simulink model "VCMGCM1962020b_v2"  (R2020b)
settings: Solver=FixedStepDiscrete  StartTime=0.0  StopTime=10.0  FixedStep=0.005  RelTol=1e-3  EnableMultiTasking=on
PreLoadFcn:
  | try, model_open; catch, disp('Error occurred while executing model pre-load callback: model_open.m'); disp('Please assure that the MATLAB working directory is set to the model directory before opening.'); end
InitFcn:
  | try, model_open; catch, end
undefined symbols (not defined in the file): Bridge, GCM, H, raptor_get_param_eval, raptor_get_safe_string, raptor_xcp_function
libraries: Blocks_lib x1165, Raptor_lib x665, simulink x62, VCM_lib x5
(part 12 of 23)

== system VCMGCM1962020b_v2/Fgnd/Sensors/CAN/Battery/Status ==
  DiagEnbl : Inport
  Bus Creator : BusCreator  Inputs=11
  CANRxField1 : Blocks_lib/CANRxField  typ='double'  custom=off  custom_nam='---'  custom_units='---'
  CANRxField{3..10} (8 alike) : Blocks_lib/CANRxField  typ='boolean'  custom=off  custom_nam='---'  custom_units='---'
  CANRxField2 : Blocks_lib/CANRxField  typ='uint8'  custom=off  custom_nam='---'  custom_units='---'
  CANRxMsgStatus : Blocks_lib/CANRxMsgStatus  samptime=samptime  custom=off  custom_nam='---'  msgnam=Status
      link override CntrSat/Constant: OutDataTypeStr=uint32
      link override CntrSat/Constant1: OutDataTypeStr=uint32
      link override CntrSat/Relational Operator: Operator=>
      link override CntrSat/raptor_adjustment: dataType=uint32
  Header : Blocks_lib/Header  width=Landscape  addtext=''
  raptor_can_rxmsg : Raptor_lib/CAN/raptor_can_rxmsg  canDefinition=struct('dbcFile', 'eMatrix_Battery.dbc','message', 'Status','comment', '','signals', {{'ActivePacks','FaultID5','FaultID4','FaultID3','FaultID2','GFD','FaultID','PreContactor','PosContactor','NegContactor'}},'enabled', [ 1 1 1 1 1 1 1 1 1 1;],'scaled', [ 1 1 1 1 1 1 1 1 1 1;],'canBus', '''CAN1''','messageID', [ 277;],'idMask', [ 536870911;],'payloadMask', [],'payloadValue', [],'period', [ 0;],'mailbox', '''''','queueSize', [ 1;],'label', [ 0;],'ver', [ 2;],'showID', [ 0;],'showRaw', [ 0;],'fill', [ 0;],'editID', [ 0;],'signalOrder', [ 3;],'signalAscDes', [ 1;])  canBus='CAN1'  mailbox=''  payloadMask=[]  payloadValue=[]  idMask=hex2dec('1FFFFFFF')  queueSize=1  showID=0  label=0  fill=0  id=277  showRaw=0  showAge=1  signalOrder=3  signalInfo={{struct('Name', 'ActivePacks','Startbit', [ 0;],'SignalSize', [ 3;],'ByteOrder', 'LittleEndian','ValueType', 'UNSIGNED','Class', 'uint8','Signed', [ 0;],'Factor', [ 1;],'Offset', [ 0;],'Min', [ 0;],'Max', [ 0;],'Units', 'nmbr','Comment', 'Number of battery packs currently connected to the HV bus.','StartBit', [ 58;]),struct('Name', 'FaultID5','Startbit', [ 0;],'SignalSize', [ 8;],'ByteOrder', 'LittleEndian','ValueType', 'UNSIGNED','Class', 'uint8','Signed', [ 0;],'Factor', [ 1;],'Offset', [ 0;],'Min', [ 0;],'Max', [ 255;],'Units', 'Enum','Comment', '','StartBit', [ 48;]),struct('Name', 'FaultID4','Startbit', [ 0;],'SignalSize', [ 8;],'ByteOrder', 'LittleEndian','ValueType', 'UNSIGNED','Class', 'uint8','Signed', [ 0;],'Factor', [ 1;],'Offset', [ 0;],'Min', [ 0;],'Max', [ 255;],'Units', 'Enum','Comment', '','StartBit', [ 40;]),struct('Name', 'FaultID3','Startbit', [ 0;],'SignalSize', [ 8;],'ByteOrder', 'LittleEndian','ValueType', 'UNSIGNED','Class', 'uint8','Signed', [ 0;],'Factor', [ 1;],'Offset', [ 0;],'Min', [ 0;],'Max', [ 255;],'Units', 'Enum','Comment', '','StartBit', [ 32;]),struct('Name', 'FaultID2','Startbit', [ 0;],'SignalSize', [ 8;],'ByteOrder', 'LittleEndian','ValueType', 'UNSIGNED','Class', 'uint8','Signed', [ 0;],'Factor', [ 1;],'Offset', [ 0;],'Min', [ 0;],'Max', [ 255;],'Units', 'Enum','Comment', '','StartBit', [ 24;]),struct('Name', 'GFD','Startbit', [ 0;],'SignalSize', [ 16;],'ByteOrder', 'LittleEndian','ValueType', 'UNSIGNED','Class', 'uint16','Signed', [ 0;],'Factor', [ 1;],'Offset', [ 0;],'Min', [ 0;],'Max', [ 0;],'Units', 'Enum','Comment', '','StartBit', [ 0;]),struct('Name', 'FaultID','Startbit', [ 0;],'SignalSize', [ 8;],'ByteOrder', 'LittleEndian','ValueType', 'UNSIGNED','Class', 'uint8','Signed', [ 0;],'Factor', [ 1;],'Offset', [ 0;],'Min', [ 0;],'Max', [ 255;],'Units', 'Enum','Comment', '','StartBit', [ 16;]),struct('Name', 'PreContactor','Startbit', [ 0;],'SignalSize', [ 1;],'ByteOrder', 'LittleEndian','ValueType', 'UNSIGNED','Class', 'uint8','Signed', [ 0;],'Factor', [ 1;],'Offset', [ 0;],'Min', [ 0;],'Max', [ 0;],'Units', 'Bool','Comment', '0 = Open','StartBit', [ 63;]),struct('Name', 'PosContactor','Startbit', [ 0;],'SignalSize', [ 1;],'ByteOrder', 'LittleEndian','ValueType', 'UNSIGNED','Class', 'uint8','Signed', [ 0;],'Factor', [ 1;],'Offset', [ 0;],'Min', [ 0;],'Max', [ 0;],'Units', 'Bool','Comment', '0 = Open','StartBit', [ 62;]),struct('Name', 'NegContactor','Startbit', [ 0;],'SignalSize', [ 1;],'ByteOrder', 'LittleEndian','ValueType', 'UNSIGNED','Class', 'uint8','Signed', [ 0;],'Factor', [ 1;],'Offset', [ 0;],'Min', [ 0;],'Max', [ 0;],'Units', 'Bool','Comment', '0 = Open','StartBit', [ 61;])}}
      settings: SourceProductName=Raptor
  Data : Outport  VectorParamsAs1DForOutWhenUnconnected=off
  wires:
  CANRxField5/1 -> Bus Creator/6
  raptor_can_rxmsg/6 -> CANRxField5/1  "Batt_FltD2"
  Bus Creator/1 -> Data/1  "Status"
  CANRxField2/1 -> Bus Creator/3
  CANRxField3/1 -> Bus Creator/4
  CANRxField4/1 -> Bus Creator/5
  raptor_can_rxmsg/2 -> CANRxField1/1  "Batt_NmbrPcksActv"
  raptor_can_rxmsg/3 -> CANRxField2/1  "Batt_FltD5"
  raptor_can_rxmsg/4 -> CANRxField3/1  "Batt_FltD4"
  raptor_can_rxmsg/5 -> CANRxField4/1  "Batt_FltD3"
  CANRxField1/1 -> Bus Creator/2
  CANRxMsgStatus/1 -> Bus Creator/1
  DiagEnbl/1 -> CANRxMsgStatus/1
  raptor_can_rxmsg/1 -> CANRxMsgStatus/2  "Age"
  raptor_can_rxmsg/7 -> CANRxField6/1  "Batt_GFD"
  raptor_can_rxmsg/8 -> CANRxField7/1  "Batt_FltD"
  raptor_can_rxmsg/9 -> CANRxField8/1  "Batt_PreCntctr"
  raptor_can_rxmsg/10 -> CANRxField9/1  "Batt_PosCntctr"
  raptor_can_rxmsg/11 -> CANRxField10/1  "Batt_NegCntctr"
  CANRxField6/1 -> Bus Creator/7
  CANRxField7/1 -> Bus Creator/8
  CANRxField8/1 -> Bus Creator/9
  CANRxField9/1 -> Bus Creator/10
  CANRxField10/1 -> Bus Creator/11

== system VCMGCM1962020b_v2/Fgnd/Sensors/CAN/CCS Interface/CCSEVSE_ChargeParameters1 ==
  DiagEnbl : Inport
  Bus Creator : BusCreator  Inputs=5
  CANRxField{,1..3} (4 alike) : Blocks_lib/CANRxField  typ='double'  custom=on  custom_nam=[nam '---']  custom_units='---'
  CANRxMsgStatus : Blocks_lib/CANRxMsgStatus  samptime=samptime  custom=on  custom_nam=[nam '---']  msgnam=CCSEVSE_ChargeParameters1
  Header : Blocks_lib/Header  width=Landscape  addtext=''
  raptor_can_rxmsg : Raptor_lib/CAN/raptor_can_rxmsg  canDefinition=struct('dbcFile', 'm2iev-api.dbc','message', 'EVSE_ChargeParameters1','comment', 'EVSE_ChargeParameters1','signals', {{'EVSEMaximumCurrentLimit','EVSEMaximumVoltageLimit','EVSEMaximumPowerLimit','EVSEEnergyToBeDelivered'}},'enabled', [ 1 1 1 1;],'canBus', 'bus','messageID', [ 514;],'idMask', [ 2047;],'payloadMask', [],'payloadValue', [],'period', [ 0;],'mailbox', '''''','queueSize', [ 1;],'label', [ 1;],'ver', [ 2;],'showID', [ 0;],'showRaw', [ 0;],'fill', [ 0;],'editID', [ 0;],'signalOrder', [ 3;])  canBus=bus  mailbox=''  payloadMask=[]  payloadValue=[]  idMask=hex2dec('7FF')  queueSize=1  showID=0  label=1  fill=0  id=514  showRaw=0  showAge=1  signalOrder=3  signalInfo={{struct('Name', 'EVSEMaximumCurrentLimit','Startbit', [ 0;],'SignalSize', [ 16;],'ByteOrder', 'LittleEndian','ValueType', 'SIGNED','Class', 'int16','Signed', [ 1;],'Factor', [ 0.05;],'Offset', [ 0;],'Min', [ -1638.4;],'Max', [ 1638.35;],'Units', 'A','Comment', 'Maximim current EVSE is able to supply','StartBit', [ 0;]),struct('Name', 'EVSEMaximumVoltageLimit','Startbit', [ 0;],'SignalSize', [ 16;],'ByteOrder', 'LittleEndian','ValueType', 'UNSIGNED','Class', 'uint16','Signed', [ 0;],'Factor', [ 0.05;],'Offset', [ 0;],'Min', [ 0;],'Max', [ 3276.75;],'Units', 'V','Comment', 'Maximim voltage EVSE is able to supply','StartBit', [ 16;]),struct('Name', 'EVSEMaximumPowerLimit','Startbit', [ 0;],'SignalSize', [ 16;],'ByteOrder', 'LittleEndian','ValueType', 'UNSIGNED','Class', 'uint16','Signed', [ 0;],'Factor', [ 0.05;],'Offset', [ 0;],'Min', [ 0;],'Max', [ 3276.75;],'Units', 'kW','Comment', 'Maximum power EVSE is able to supply','StartBit', [ 32;]),struct('Name', 'EVSEEnergyToBeDelivered','Startbit', [ 0;],'SignalSize', [ 16;],'ByteOrder', 'LittleEndian','ValueType', 'UNSIGNED','Class', 'uint16','Signed', [ 0;],'Factor', [ 0.05;],'Offset', [ 0;],'Min', [ 0;],'Max', [ 3276.75;],'Units', 'kWh','Comment', 'Approximation of energy to be delivered','StartBit', [ 48;])}}
      settings: SourceProductName=Raptor
  Data : Outport  VectorParamsAs1DForOutWhenUnconnected=off
  wires:
  Bus Creator/1 -> Data/1  "MsgName"
  raptor_can_rxmsg/2 -> CANRxField/1  "EVSEMaximumCurrentLimit"
  raptor_can_rxmsg/3 -> CANRxField1/1  "EVSEMaximumVoltageLimit"
  raptor_can_rxmsg/4 -> CANRxField2/1  "EVSEMaximumPowerLimit"
  raptor_can_rxmsg/5 -> CANRxField3/1  "EVSEEnergyToBeDelivered"
  CANRxField3/1 -> Bus Creator/5
  CANRxField2/1 -> Bus Creator/4
  CANRxField1/1 -> Bus Creator/3
  CANRxField/1 -> Bus Creator/2
  CANRxMsgStatus/1 -> Bus Creator/1
  DiagEnbl/1 -> CANRxMsgStatus/1
  raptor_can_rxmsg/1 -> CANRxMsgStatus/2  "Age"

== system VCMGCM1962020b_v2/Fgnd/Sensors/CAN/CCS Interface/CCSEVSE_ChargeParameters2 ==
  DiagEnbl : Inport
  Bus Creator : BusCreator  Inputs=5
  CANRxField{,1..3} (4 alike) : Blocks_lib/CANRxField  typ='double'  custom=on  custom_nam=[nam '---']  custom_units='---'
  CANRxMsgStatus : Blocks_lib/CANRxMsgStatus  samptime=samptime  custom=on  custom_nam=[nam '---']  msgnam=CCSEVSE_ChargeParameters2
  Header : Blocks_lib/Header  width=Landscape  addtext=''
  raptor_can_rxmsg : Raptor_lib/CAN/raptor_can_rxmsg  canDefinition=struct('dbcFile', 'm2iev-api.dbc','message', 'EVSE_ChargeParameters2','comment', 'EVSE_ChargeParameters2','signals', {{'EVSEMinimumCurrentLimit','EVSEMinimumVoltageLimit','EVSECurrentRegulationTolerance','EVSEPeakCurrentRipple'}},'enabled', [ 1 1 1 1;],'canBus', 'bus','messageID', [ 515;],'idMask', [ 2047;],'payloadMask', [],'payloadValue', [],'period', [ 0;],'mailbox', '''''','queueSize', [ 1;],'label', [ 1;],'ver', [ 2;],'showID', [ 0;],'showRaw', [ 0;],'fill', [ 0;],'editID', [ 0;],'signalOrder', [ 3;])  canBus=bus  mailbox=''  payloadMask=[]  payloadValue=[]  idMask=hex2dec('7FF')  queueSize=1  showID=0  label=1  fill=0  id=515  showRaw=0  showAge=1  signalOrder=3  signalInfo={{struct('Name', 'EVSEMinimumCurrentLimit','Startbit', [ 0;],'SignalSize', [ 16;],'ByteOrder', 'LittleEndian','ValueType', 'SIGNED','Class', 'int16','Signed', [ 1;],'Factor', [ 0.05;],'Offset', [ 0;],'Min', [ -1638.4;],'Max', [ 1638.35;],'Units', 'A','Comment', 'Minimum current EVSE is able to supply','StartBit', [ 0;]),struct('Name', 'EVSEMinimumVoltageLimit','Startbit', [ 0;],'SignalSize', [ 16;],'ByteOrder', 'LittleEndian','ValueType', 'UNSIGNED','Class', 'uint16','Signed', [ 0;],'Factor', [ 0.05;],'Offset', [ 0;],'Min', [ 0;],'Max', [ 3276.75;],'Units', 'V','Comment', 'Minimum voltage EVSE is able to supply','StartBit', [ 16;]),struct('Name', 'EVSECurrentRegulationTolerance','Startbit', [ 0;],'SignalSize', [ 8;],'ByteOrder', 'LittleEndian','ValueType', 'UNSIGNED','Class', 'uint8','Signed', [ 0;],'Factor', [ 0.5;],'Offset', [ 0;],'Min', [ 0;],'Max', [ 127.5;],'Units', 'A','Comment', 'Tolerance of the current regulation','StartBit', [ 32;]),struct('Name', 'EVSEPeakCurrentRipple','Startbit', [ 0;],'SignalSize', [ 8;],'ByteOrder', 'LittleEndian','ValueType', 'UNSIGNED','Class', 'uint8','Signed', [ 0;],'Factor', [ 0.5;],'Offset', [ 0;],'Min', [ 0;],'Max', [ 127.5;],'Units', 'A','Comment', 'Peak current ripple that may occur on EVSE output','StartBit', [ 40;])}}
      settings: SourceProductName=Raptor
  Data : Outport  VectorParamsAs1DForOutWhenUnconnected=off
  wires:
  raptor_can_rxmsg/5 -> CANRxField3/1  "EVSEPeakCurrentRipple"
  raptor_can_rxmsg/4 -> CANRxField2/1  "EVSECurrentRegulationTolerance"
  raptor_can_rxmsg/3 -> CANRxField1/1  "EVSEMinimumVoltageLimit"
  raptor_can_rxmsg/2 -> CANRxField/1  "EVSEMinimumCurrentLimit"
  Bus Creator/1 -> Data/1  "MsgName"
  CANRxField3/1 -> Bus Creator/5
  CANRxField2/1 -> Bus Creator/4
  CANRxField1/1 -> Bus Creator/3
  CANRxField/1 -> Bus Creator/2
  CANRxMsgStatus/1 -> Bus Creator/1
  DiagEnbl/1 -> CANRxMsgStatus/1
  raptor_can_rxmsg/1 -> CANRxMsgStatus/2  "Age"

== system VCMGCM1962020b_v2/Fgnd/Sensors/CAN/CCS Interface/CCSEVSE_DC_ChargeInfo1 ==
  DiagEnbl : Inport
  Bus Creator : BusCreator  Inputs=9
  CANRxField : Blocks_lib/CANRxField  typ='uint8'  custom=on  custom_nam=[nam '---']  custom_units='---'
  CANRxField1 : Blocks_lib/CANRxField  typ='boolean'  custom=on  custom_nam=[nam '---']  custom_units='---'
  CANRxField2 : Blocks_lib/CANRxField  typ='boolean'  custom=on  custom_nam=[nam '---']  custom_units='---'
  CANRxField3 : Blocks_lib/CANRxField  typ='boolean'  custom=on  custom_nam=[nam '---']  custom_units='---'
  CANRxField4 : Blocks_lib/CANRxField  typ='uint8'  custom=on  custom_nam=[nam '---']  custom_units='---'
  CANRxField5 : Blocks_lib/CANRxField  typ='uint8'  custom=on  custom_nam=[nam '---']  custom_units='---'
  CANRxField6 : Blocks_lib/CANRxField  typ='double'  custom=on  custom_nam=[nam '---']  custom_units='---'
  CANRxField7 : Blocks_lib/CANRxField  typ='double'  custom=on  custom_nam=[nam '---']  custom_units='---'
  CANRxMsgStatus : Blocks_lib/CANRxMsgStatus  samptime=samptime  custom=on  custom_nam=[nam '---']  msgnam=CCSEVSE_DC_ChargeInfo1
  Header : Blocks_lib/Header  width=Landscape  addtext=''
  raptor_can_rxmsg : Raptor_lib/CAN/raptor_can_rxmsg  canDefinition=struct('dbcFile', 'm2iev-api.dbc','message', 'EVSE_DC_ChargeInfo1','comment', 'EVSE_DC_ChargeInfo1','signals', {{'ResponseCode','EVSECurrentLimitAchieved','EVSEVoltageLimitAchieved','EVSEPowerLimitAchieved','EVSEStatusCode','EVSEIsolationStatus','EVSEPresentVoltage','EVSEPresentCurrent'}},'enabled', [ 1 1 1 1 1 1 1 1;],'canBus', 'bus','messageID', [ 257;],'idMask', [ 2047;],'payloadMask', [],'payloadValue', [],'period', [ 0;],'mailbox', '''''','queueSize', [ 1;],'label', [ 1;],'ver', [ 2;],'showID', [ 0;],'showRaw', [ 0;],'fill', [ 0;],'editID', [ 0;],'signalOrder', [ 3;])  canBus=bus  mailbox=''  payloadMask=[]  payloadValue=[]  idMask=hex2dec('7FF')  queueSize=1  showID=0  label=1  fill=0  id=257  showRaw=0  showAge=1  signalOrder=3  signalInfo={{struct('Name', 'ResponseCode','Startbit', [ 0;],'SignalSize', [ 5;],'ByteOrder', 'LittleEndian','ValueType', 'UNSIGNED','Class', 'uint8','Signed', [ 0;],'Factor', [ 1;],'Offset', [ 0;],'Min', [ 0;],'Max', [ 26;],'Units', 'Enum','Comment', 'Response code from EVSE','StartBit', [ 0;]),struct('Name', 'EVSECurrentLimitAchieved','Startbit', [ 0;],'SignalSize', [ 1;],'ByteOrder', 'LittleEndian','ValueType', 'UNSIGNED','Class', 'uint8','Signed', [ 0;],'Factor', [ 1;],'Offset', [ 0;],'Min', [ 0;],'Max', [ 1;],'Units', 'Boolean','Comment', 'Indicator that EVSE is in current limiting mode','StartBit', [ 5;]),struct('Name', 'EVSEVoltageLimitAchieved','Startbit', [ 0;],'SignalSize', [ 1;],'ByteOrder', 'LittleEndian','ValueType', 'UNSIGNED','Class', 'uint8','Signed', [ 0;],'Factor', [ 1;],'Offset', [ 0;],'Min', [ 0;],'Max', [ 1;],'Units', 'Boolean','Comment', 'Indicator that EVSE is in voltage limiting mode','StartBit', [ 6;]),struct('Name', 'EVSEPowerLimitAchieved','Startbit', [ 0;],'SignalSize', [ 1;],'ByteOrder', 'LittleEndian','ValueType', 'UNSIGNED','Class', 'uint8','Signed', [ 0;],'Factor', [ 1;],'Offset', [ 0;],'Min', [ 0;],'Max', [ 1;],'Units', 'Boolean','Comment', 'Indicator that EVSE is in power limiting mode','StartBit', [ 7;]),struct('Name', 'EVSEStatusCode','Startbit', [ 0;],'SignalSize', [ 4;],'ByteOrder', 'LittleEndian','ValueType', 'UNSIGNED','Class', 'uint8','Signed', [ 0;],'Factor', [ 1;],'Offset', [ 0;],'Min', [ 0;],'Max', [ 11;],'Units', 'Enum','Comment', 'Status code reported by EVSE','StartBit', [ 8;]),struct('Name', 'EVSEIsolationStatus','Startbit', [ 0;],'SignalSize', [ 2;],'ByteOrder', 'LittleEndian','ValueType', 'UNSIGNED','Class', 'uint8','Signed', [ 0;],'Factor', [ 1;],'Offset', [ 0;],'Min', [ 0;],'Max', [ 3;],'Units', 'Enum','Comment', 'Isolation status detected by EVSE','StartBit', [ 12;]),struct('Name', 'EVSEPresentVoltage','Startbit', [ 0;],'SignalSize', [ 16;],'ByteOrder', 'LittleEndian','ValueType', 'UNSIGNED','Class', 'uint16','Signed', [ 0;],'Factor', [ 0.05;],'Offset', [ 0;],'Min', [ 0;],'Max', [ 3276.75;],'Units', 'V','Comment', 'Voltage supplied by EVSE (read on EVSE side)','StartBit', [ 16;]),struct('Name', 'EVSEPresentCurrent','Startbit', [ 0;],'SignalSize', [ 16;],'ByteOrder', 'LittleEndian','ValueType', 'SIGNED','Class', 'int16','Signed', [ 1;],'Factor', [ 0.05;],'Offset', [ 0;],'Min', [ -1638.4;],'Max', [ 1638.35;],'Units', 'A','Comment', 'Current supplied by EVSE (read on EVSE side)','StartBit', [ 32;])}}
      settings: SourceProductName=Raptor
  Data : Outport  VectorParamsAs1DForOutWhenUnconnected=off
  wires:
  raptor_can_rxmsg/6 -> CANRxField4/1  "EVSEStatusCode"
  raptor_can_rxmsg/5 -> CANRxField3/1  "EVSEPowerLimitAchieved"
  raptor_can_rxmsg/4 -> CANRxField2/1  "EVSEVoltageLimitAchieved"
  raptor_can_rxmsg/3 -> CANRxField1/1  "EVSECurrentLimitAchieved"
  raptor_can_rxmsg/2 -> CANRxField/1  "ResponseCode"
  Bus Creator/1 -> Data/1  "MsgName"
  raptor_can_rxmsg/7 -> CANRxField5/1  "EVSEIsolationStatus"
  raptor_can_rxmsg/8 -> CANRxField6/1  "EVSEPresentVoltage"
  raptor_can_rxmsg/9 -> CANRxField7/1  "EVSEPresentCurrent"
  CANRxField7/1 -> Bus Creator/9
  CANRxField6/1 -> Bus Creator/8
  CANRxField5/1 -> Bus Creator/7
  CANRxField4/1 -> Bus Creator/6
  CANRxField3/1 -> Bus Creator/5
  CANRxField2/1 -> Bus Creator/4
  CANRxField1/1 -> Bus Creator/3
  CANRxField/1 -> Bus Creator/2
  CANRxMsgStatus/1 -> Bus Creator/1
  DiagEnbl/1 -> CANRxMsgStatus/1
  raptor_can_rxmsg/1 -> CANRxMsgStatus/2  "Age"

== system VCMGCM1962020b_v2/Fgnd/Sensors/CAN/CCS Interface/CCSM2IEV_Alerts ==
  DiagEnbl : Inport
  Bus Creator : BusCreator  Inputs=16
  CANRxField{,1..14} (15 alike) : Blocks_lib/CANRxField  typ='boolean'  custom=on  custom_nam=[nam '---']  custom_units='---'
  CANRxMsgStatus : Blocks_lib/CANRxMsgStatus  samptime=samptime  custom=on  custom_nam=[nam '---']  msgnam=CCSM2IEV_Alerts
  Header : Blocks_lib/Header  width=Landscape  addtext=''
  raptor_can_rxmsg : Raptor_lib/CAN/raptor_can_rxmsg  canDefinition=struct('dbcFile', 'm2iev-api.dbc','message', 'M2IEV_Alerts','comment', 'M2IEV_Alerts','signals', {{'TemperatureDC1HighAlarm','TemperatureDC1HighFault','TemperatureDC1LowAlarm','TemperatureDC1LowFault','TemperatureDC2HighAlarm','TemperatureDC2HighFault','TemperatureDC2LowAlarm','TemperatureDC2LowFault','TemperatureACFault','EmergencyStopFault','PilotFault','ProximityFault','CanRxFault','SocketLatchSensorFault','EvccError'}},'enabled', [ 1 1 1 1 1 1 1 1 1 1 1 1 1 1 1;],'canBus', 'bus','messageID', [ 260;],'idMask', [ 2047;],'payloadMask', [],'payloadValue', [],'period', [ 0;],'mailbox', '''''','queueSize', [ 1;],'label', [ 1;],'ver', [ 2;],'showID', [ 0;],'showRaw', [ 0;],'fill', [ 0;],'editID', [ 0;],'signalOrder', [ 3;],'signalAscDes', [ 1;])  canBus=bus  mailbox=''  payloadMask=[]  payloadValue=[]  idMask=hex2dec('7FF')  queueSize=1  showID=0  label=1  fill=0  id=260  showRaw=0  showAge=1  signalOrder=3  signalInfo={{struct('Name', 'TemperatureDC1HighAlarm','Startbit', [ 0;],'SignalSize', [ 1;],'ByteOrder', 'LittleEndian','ValueType', 'UNSIGNED','Class', 'uint8','Signed', [ 0;],'Factor', [ 1;],'Offset', [ 0;],'Min', [ 0;],'Max', [ 1;],'Units', 'Boolean','Comment', 'Temperature on DC+ terminal >=80 degC','StartBit', [ 0;]),struct('Name', 'TemperatureDC1HighFault','Startbit', [ 0;],'SignalSize', [ 1;],'ByteOrder', 'LittleEndian','ValueType', 'UNSIGNED','Class', 'uint8','Signed', [ 0;],'Factor', [ 1;],'Offset', [ 0;],'Min', [ 0;],'Max', [ 1;],'Units', 'Boolean','Comment', 'Temperature on DC+ terminal >=90 degC','StartBit', [ 1;]),struct('Name', 'TemperatureDC1LowAlarm','Startbit', [ 0;],'SignalSize', [ 1;],'ByteOrder', 'LittleEndian','ValueType', 'UNSIGNED','Class', 'uint8','Signed', [ 0;],'Factor', [ 1;],'Offset', [ 0;],'Min', [ 0;],'Max', [ 1;],'Units', 'Boolean','Comment', 'Temperature on DC+ terminal <=-20 degC','StartBit', [ 2;]),struct('Name', 'TemperatureDC1LowFault','Startbit', [ 0;],'SignalSize', [ 1;],'ByteOrder', 'LittleEndian','ValueType', 'UNSIGNED','Class', 'uint8','Signed', [ 0;],'Factor', [ 1;],'Offset', [ 0;],'Min', [ 0;],'Max', [ 1;],'Units', 'Boolean','Comment', 'Temperature on DC+ terminal <=-30 degC','StartBit', [ 3;]),struct('Name', 'TemperatureDC2HighAlarm','Startbit', [ 0;],'SignalSize', [ 1;],'ByteOrder', 'LittleEndian','ValueType', 'UNSIGNED','Class', 'uint8','Signed', [ 0;],'Factor', [ 1;],'Offset', [ 0;],'Min', [ 0;],'Max', [ 1;],'Units', 'Boolean','Comment', 'Temperature on DC- terminal >=80 degC','StartBit', [ 4;]),struct('Name', 'TemperatureDC2HighFault','Startbit', [ 0;],'SignalSize', [ 1;],'ByteOrder', 'LittleEndian','ValueType', 'UNSIGNED','Class', 'uint8','Signed', [ 0;],'Factor', [ 1;],'Offset', [ 0;],'Min', [ 0;],'Max', [ 1;],'Units', 'Boolean','Comment', 'Temperature on DC- terminal >=90 degC','StartBit', [ 5;]),struct('Name', 'TemperatureDC2LowAlarm','Startbit', [ 0;],'SignalSize', [ 1;],'ByteOrder', 'LittleEndian','ValueType', 'UNSIGNED','Class', 'uint8','Signed', [ 0;],'Factor', [ 1;],'Offset', [ 0;],'Min', [ 0;],'Max', [ 1;],'Units', 'Boolean','Comment', 'Temperature on DC- terminal <=-20 degC','StartBit', [ 6;]),struct('Name', 'TemperatureDC2LowFault','Startbit', [ 0;],'SignalSize', [ 1;],'ByteOrder', 'LittleEndian','ValueType', 'UNSIGNED','Class', 'uint8','Signed', [ 0;],'Factor', [ 1;],'Offset', [ 0;],'Min', [ 0;],'Max', [ 1;],'Units', 'Boolean','Comment', 'Temperature on DC- terminal <=-30 degC','StartBit', [ 7;]),struct('Name', 'TemperatureACFault','Startbit', [ 0;],'SignalSize', [ 1;],'ByteOrder', 'LittleEndian','ValueType', 'UNSIGNED','Class', 'uint8','Signed', [ 0;],'Factor', [ 1;],'Offset', [ 0;],'Min', [ 0;],'Max', [ 1;],'Units', 'Boolean','Comment', 'Temperature on AC terminals is too high','StartBit', [ 8;]),struct('Name', 'EmergencyStopFault','Startbit', [ 0;],'SignalSize', [ 1;],'ByteOrder', 'LittleEndian','ValueType', 'UNSIGNED','Class', 'uint8','Signed', [ 0;],'Factor', [ 1;],'Offset', [ 0;],'Min', [ 0;],'Max', [ 1;],'Units', 'Boolean','Comment', 'Emergency stop','StartBit', [ 9;]),struct('Name', 'PilotFault','Startbit', [ 0;],'SignalSize', [ 1;],'ByteOrder', 'LittleEndian','ValueType', 'UNSIGNED','Class', 'uint8','Signed', [ 0;],'Factor', [ 1;],'Offset', [ 0;],'Min', [ 0;],'Max', [ 1;],'Units', 'Boolean','Comment', 'Pilot fault','StartBit', [ 10;]),struct('Name', 'ProximityFault','Startbit', [ 0;],'SignalSize', [ 1;],'ByteOrder', 'LittleEndian','ValueType', 'UNSIGNED','Class', 'uint8','Signed', [ 0;],'Factor', [ 1;],'Offset', [ 0;],'Min', [ 0;],'Max', [ 1;],'Units', 'Boolean','Comment', 'Proximity fault','StartBit', [ 11;]),struct('Name', 'CanRxFault','Startbit', [ 0;],'SignalSize', [ 1;],'ByteOrder', 'LittleEndian','ValueType', 'UNSIGNED','Class', 'uint8','Signed', [ 0;],'Factor', [ 1;],'Offset', [ 0;],'Min', [ 0;],'Max', [ 1;],'Units', 'Boolean','Comment', 'Can Rx fault','StartBit', [ 12;]),struct('Name', 'SocketLatchSensorFault','Startbit', [ 0;],'SignalSize', [ 1;],'ByteOrder', 'LittleEndian','ValueType', 'UNSIGNED','Class', 'uint8','Signed', [ 0;],'Factor', [ 1;],'Offset', [ 0;],'Min', [ 0;],'Max', [ 1;],'Units', 'Boolean','Comment', 'Socket latch sensor fault','StartBit', [ 13;]),struct('Name', 'EvccError','Startbit', [ 0;],'SignalSize', [ 1;],'ByteOrder', 'LittleEndian','ValueType', 'UNSIGNED','Class', 'uint8','Signed', [ 0;],'Factor', [ 1;],'Offset', [ 0;],'Min', [ 0;],'Max', [ 1;],'Units', 'Boolean','Comment', 'Received EVCC error','StartBit', [ 14;])}}
      settings: SourceProductName=Raptor
  Data : Outport  VectorParamsAs1DForOutWhenUnconnected=off
  wires:
  raptor_can_rxmsg/10 -> CANRxField8/1  "TemperatureACFault"
  raptor_can_rxmsg/11 -> CANRxField9/1  "EmergencyStopFault"
  raptor_can_rxmsg/13 -> CANRxField11/1  "ProximityFault"
  raptor_can_rxmsg/12 -> CANRxField10/1  "PilotFault"
  raptor_can_rxmsg/16 -> CANRxField14/1  "EvccError"
  raptor_can_rxmsg/15 -> CANRxField13/1  "SocketLatchSensorFault"
  raptor_can_rxmsg/14 -> CANRxField12/1  "CanRxFault"
  raptor_can_rxmsg/6 -> CANRxField4/1  "TemperatureDC2HighAlarm"
  raptor_can_rxmsg/7 -> CANRxField5/1  "TemperatureDC2HighFault"
  raptor_can_rxmsg/9 -> CANRxField7/1  "TemperatureDC2LowFault"
  raptor_can_rxmsg/8 -> CANRxField6/1  "TemperatureDC2LowAlarm"
  raptor_can_rxmsg/4 -> CANRxField2/1  "TemperatureDC1LowAlarm"
  raptor_can_rxmsg/5 -> CANRxField3/1  "TemperatureDC1LowFault"
  raptor_can_rxmsg/3 -> CANRxField1/1  "TemperatureDC1HighFault"
  raptor_can_rxmsg/2 -> CANRxField/1  "TemperatureDC1HighAlarm"
  Bus Creator/1 -> Data/1  "MsgName"
  CANRxField11/1 -> Bus Creator/13
  CANRxField10/1 -> Bus Creator/12
  CANRxField12/1 -> Bus Creator/14
  CANRxField9/1 -> Bus Creator/11
  CANRxField13/1 -> Bus Creator/15
  CANRxField8/1 -> Bus Creator/10
  CANRxField14/1 -> Bus Creator/16
  CANRxField7/1 -> Bus Creator/9
  CANRxField6/1 -> Bus Creator/8
  CANRxField5/1 -> Bus Creator/7
  CANRxField4/1 -> Bus Creator/6
  CANRxField3/1 -> Bus Creator/5
  CANRxField2/1 -> Bus Creator/4
  CANRxField1/1 -> Bus Creator/3
  CANRxField/1 -> Bus Creator/2
  CANRxMsgStatus/1 -> Bus Creator/1
  DiagEnbl/1 -> CANRxMsgStatus/1
  raptor_can_rxmsg/1 -> CANRxMsgStatus/2  "Age"

== system VCMGCM1962020b_v2/Fgnd/Sensors/CAN/CCS Interface/CCSM2IEV_Command ==
  DiagEnbl : Inport
  Bus Creator : BusCreator  Inputs=8
  CANRxField{,1,5..6} (4 alike) : Blocks_lib/CANRxField  typ='uint8'  custom=on  custom_nam=[nam '---']  custom_units='---'
  CANRxField2 : Blocks_lib/CANRxField  typ='boolean'  custom=on  custom_nam=[nam '---']  custom_units='---'
  CANRxField3 : Blocks_lib/CANRxField  typ='boolean'  custom=on  custom_nam=[nam '---']  custom_units='---'
  CANRxField4 : Blocks_lib/CANRxField  typ='boolean'  custom=on  custom_nam=[nam '---']  custom_units='---'
  CANRxMsgStatus : Blocks_lib/CANRxMsgStatus  samptime=samptime  custom=on  custom_nam=[nam '---']  msgnam=CCSM2IEV_Command
  Header : Blocks_lib/Header  width=Landscape  addtext=''
  raptor_can_rxmsg : Raptor_lib/CAN/raptor_can_rxmsg  canDefinition=struct('dbcFile', 'm2iev-api.dbc','message', 'M2IEV_Command','comment', 'M2IEV_Command','signals', {{'CurrentState','ChargerType','AC_CloseContactorsRequest','DC_CloseContactorsRequest','PrechargeReady','SocketLockState','ErrorCode'}},'enabled', [ 1 1 1 1 1 1 1;],'canBus', 'bus','messageID', [ 129;],'idMask', [ 2047;],'payloadMask', [],'payloadValue', [],'period', [ 0;],'mailbox', '''''','queueSize', [ 1;],'label', [ 1;],'ver', [ 2;],'showID', [ 0;],'showRaw', [ 0;],'fill', [ 0;],'editID', [ 0;],'signalOrder', [ 3;])  canBus=bus  mailbox=''  payloadMask=[]  payloadValue=[]  idMask=hex2dec('7FF')  queueSize=1  showID=0  label=1  fill=0  id=129  showRaw=0  showAge=1  signalOrder=3  signalInfo={{struct('Name', 'CurrentState','Startbit', [ 0;],'SignalSize', [ 8;],'ByteOrder', 'LittleEndian','ValueType', 'UNSIGNED','Class', 'uint8','Signed', [ 0;],'Factor', [ 1;],'Offset', [ 0;],'Min', [ 0;],'Max', [ 255;],'Units', 'Enum','Comment', 'Current state of M2IEV module','StartBit', [ 0;]),struct('Name', 'ChargerType','Startbit', [ 0;],'SignalSize', [ 3;],'ByteOrder', 'LittleEndian','ValueType', 'UNSIGNED','Class', 'uint8','Signed', [ 0;],'Factor', [ 1;],'Offset', [ 0;],'Min', [ 0;],'Max', [ 3;],'Units', 'Enum','Comment', 'Type of the charger connected','StartBit', [ 8;]),struct('Name', 'AC_CloseContactorsRequest','Startbit', [ 0;],'SignalSize', [ 1;],'ByteOrder', 'LittleEndian','ValueType', 'UNSIGNED','Class', 'uint8','Signed', [ 0;],'Factor', [ 1;],'Offset', [ 0;],'Min', [ 0;],'Max', [ 1;],'Units', 'Boolean','Comment', 'Request to close AC contactors (i.e. request to start power transfer)','StartBit', [ 11;]),struct('Name', 'DC_CloseContactorsRequest','Startbit', [ 0;],'SignalSize', [ 1;],'ByteOrder', 'LittleEndian','ValueType', 'UNSIGNED','Class', 'uint8','Signed', [ 0;],'Factor', [ 1;],'Offset', [ 0;],'Min', [ 0;],'Max', [ 1;],'Units', 'Boolean','Comment', 'Request to close DC contactors (i.e. request to start power transfer)','StartBit', [ 12;]),struct('Name', 'PrechargeReady','Startbit', [ 0;],'SignalSize', [ 1;],'ByteOrder', 'LittleEndian','ValueType', 'UNSIGNED','Class', 'uint8','Signed', [ 0;],'Factor', [ 1;],'Offset', [ 0;],'Min', [ 0;],'Max', [ 1;],'Units', 'Boolean','Comment', 'Indicator that cable check has successfully passed and we are ready to start precharging (valid only in case of smart DC charging)','StartBit', [ 13;]),struct('Name', 'SocketLockState','Startbit', [ 0;],'SignalSize', [ 3;],'ByteOrder', 'LittleEndian','ValueType', 'UNSIGNED','Class', 'uint8','Signed', [ 0;],'Factor', [ 1;],'Offset', [ 0;],'Min', [ 0;],'Max', [ 5;],'Units', 'Enum','Comment', 'Current socket state','StartBit', [ 24;]),struct('Name', 'ErrorCode','Startbit', [ 0;],'SignalSize', [ 16;],'ByteOrder', 'LittleEndian','ValueType', 'UNSIGNED','Class', 'uint16','Signed', [ 0;],'Factor', [ 1;],'Offset', [ 0;],'Min', [ 0;],'Max', [ 65535;],'Units', 'Enum','Comment', 'Internal M2IEV or EVCC error code','StartBit', [ 32;])}}
      settings: SourceProductName=Raptor
  Data : Outport  VectorParamsAs1DForOutWhenUnconnected=off
  wires:
  raptor_can_rxmsg/6 -> CANRxField4/1  "PrechargeReady"
  raptor_can_rxmsg/5 -> CANRxField3/1  "DC_CloseContactorsRequest"
  raptor_can_rxmsg/4 -> CANRxField2/1  "AC_CloseContactorsRequest"
  raptor_can_rxmsg/3 -> CANRxField1/1  "ChargerType"
  raptor_can_rxmsg/2 -> CANRxField/1  "CurrentState"
  Bus Creator/1 -> Data/1  "MsgName"
  raptor_can_rxmsg/7 -> CANRxField5/1  "SocketLockState"
  raptor_can_rxmsg/8 -> CANRxField6/1  "ErrorCode"
  CANRxField6/1 -> Bus Creator/8
  CANRxField5/1 -> Bus Creator/7
  CANRxField4/1 -> Bus Creator/6
  CANRxField3/1 -> Bus Creator/5
  CANRxField2/1 -> Bus Creator/4
  CANRxField1/1 -> Bus Creator/3
  CANRxField/1 -> Bus Creator/2
  CANRxMsgStatus/1 -> Bus Creator/1
  DiagEnbl/1 -> CANRxMsgStatus/1
  raptor_can_rxmsg/1 -> CANRxMsgStatus/2  "Age"

== system VCMGCM1962020b_v2/Fgnd/Sensors/CAN/CCS Interface/CCSM2IEV_Info ==
  DiagEnbl : Inport
  Bus Creator : BusCreator  Inputs=5
  CANRxField : Blocks_lib/CANRxField  typ='uint8'  custom=on  custom_nam=[nam '---']  custom_units='---'
  CANRxField1 : Blocks_lib/CANRxField  typ='uint8'  custom=on  custom_nam=[nam '---']  custom_units='---'
  CANRxField2 : Blocks_lib/CANRxField  typ='double'  custom=on  custom_nam=[nam '---']  custom_units='---'
  CANRxField3 : Blocks_lib/CANRxField  typ='double'  custom=on  custom_nam=[nam '---']  custom_units='---'
  CANRxMsgStatus : Blocks_lib/CANRxMsgStatus  samptime=samptime  custom=on  custom_nam=[nam '---']  msgnam=CCSM2IEV_Info
  Header : Blocks_lib/Header  width=Landscape  addtext=''
  raptor_can_rxmsg : Raptor_lib/CAN/raptor_can_rxmsg  canDefinition=struct('dbcFile', 'm2iev-api.dbc','message', 'M2IEV_Info','comment', 'M2IEV_Info','signals', {{'PP_State','CP_State','CP_PWM','CP_Voltage'}},'enabled', [ 1 1 1 1;],'canBus', 'bus','messageID', [ 130;],'idMask', [ 2047;],'payloadMask', [],'payloadValue', [],'period', [ 0;],'mailbox', '''''','queueSize', [ 1;],'label', [ 1;],'ver', [ 2;],'showID', [ 0;],'showRaw', [ 0;],'fill', [ 0;],'editID', [ 0;],'signalOrder', [ 3;],'signalAscDes', [ 1;])  canBus=bus  mailbox=''  payloadMask=[]  payloadValue=[]  idMask=hex2dec('7FF')  queueSize=1  showID=0  label=1  fill=0  id=130  showRaw=0  showAge=1  signalOrder=3  signalInfo={{struct('Name', 'PP_State','Startbit', [ 0;],'SignalSize', [ 4;],'ByteOrder', 'LittleEndian','ValueType', 'UNSIGNED','Class', 'uint8','Signed', [ 0;],'Factor', [ 1;],'Offset', [ 0;],'Min', [ 0;],'Max', [ 7;],'Units', 'Enum','Comment', 'Current proximity state','StartBit', [ 0;]),struct('Name', 'CP_State','Startbit', [ 0;],'SignalSize', [ 4;],'ByteOrder', 'LittleEndian','ValueType', 'UNSIGNED','Class', 'uint8','Signed', [ 0;],'Factor', [ 1;],'Offset', [ 0;],'Min', [ 0;],'Max', [ 7;],'Units', 'Enum','Comment', 'Current control pilot state','StartBit', [ 4;]),struct('Name', 'CP_PWM','Startbit', [ 0;],'SignalSize', [ 8;],'ByteOrder', 'LittleEndian','ValueType', 'UNSIGNED','Class', 'uint8','Signed', [ 0;],'Factor', [ 1;],'Offset', [ 0;],'Min', [ 0;],'Max', [ 100;],'Units', '%','Comment', 'Current control pilot PWM duty ratio','StartBit', [ 8;]),struct('Name', 'CP_Voltage','Startbit', [ 0;],'SignalSize', [ 9;],'ByteOrder', 'LittleEndian','ValueType', 'SIGNED','Class', 'int16','Signed', [ 1;],'Factor', [ 0.1;],'Offset', [ 0;],'Min', [ -25.6;],'Max', [ 25.5;],'Units', 'V','Comment', 'Current voltage on control pilot line','StartBit', [ 16;])}}
      settings: SourceProductName=Raptor
  Data : Outport  VectorParamsAs1DForOutWhenUnconnected=off
  wires:
  raptor_can_rxmsg/5 -> CANRxField3/1  "CP_Voltage"
  raptor_can_rxmsg/4 -> CANRxField2/1  "CP_PWM"
  raptor_can_rxmsg/3 -> CANRxField1/1  "CP_State"
  raptor_can_rxmsg/2 -> CANRxField/1  "PP_State"
  Bus Creator/1 -> Data/1  "MsgName"
  CANRxField3/1 -> Bus Creator/5
  CANRxField2/1 -> Bus Creator/4
  CANRxField1/1 -> Bus Creator/3
  CANRxField/1 -> Bus Creator/2
  CANRxMsgStatus/1 -> Bus Creator/1
  DiagEnbl/1 -> CANRxMsgStatus/1
  raptor_can_rxmsg/1 -> CANRxMsgStatus/2  "Age"

== system VCMGCM1962020b_v2/Fgnd/Sensors/CAN/CCS Interface/CCSM2IEV_TemperatureInfo ==
  DiagEnbl : Inport
  Bus Creator : BusCreator  Inputs=4
  CANRxField : Blocks_lib/CANRxField  typ='double'  custom=on  custom_nam=[nam '---']  custom_units='---'
  CANRxField1 : Blocks_lib/CANRxField  typ='double'  custom=on  custom_nam=[nam '---']  custom_units='---'
  CANRxField2 : Blocks_lib/CANRxField  typ='double'  custom=on  custom_nam=[nam '---']  custom_units='---'
  CANRxMsgStatus : Blocks_lib/CANRxMsgStatus  samptime=samptime  custom=on  custom_nam=[nam '---']  msgnam=CCSM2IEV_TemperatureInfo
  Header : Blocks_lib/Header  width=Landscape  addtext=''
  raptor_can_rxmsg : Raptor_lib/CAN/raptor_can_rxmsg  canDefinition=struct('dbcFile', 'm2iev-api.dbc','message', 'M2IEV_TemperatureInfo','comment', 'M2IEV_TemperatureInfo','signals', {{'TemperatureDC1','TemperatureDC2','TemperatureAC'}},'enabled', [ 1 1 1;],'canBus', 'bus','messageID', [ 768;],'idMask', [ 2047;],'payloadMask', [],'payloadValue', [],'period', [ 0;],'mailbox', '''''','queueSize', [ 1;],'label', [ 1;],'ver', [ 2;],'showID', [ 0;],'showRaw', [ 0;],'fill', [ 0;],'editID', [ 0;],'signalOrder', [ 3;])  canBus=bus  mailbox=''  payloadMask=[]  payloadValue=[]  idMask=hex2dec('7FF')  queueSize=1  showID=0  label=1  fill=0  id=768  showRaw=0  showAge=1  signalOrder=3  signalInfo={{struct('Name', 'TemperatureDC1','Startbit', [ 0;],'SignalSize', [ 16;],'ByteOrder', 'LittleEndian','ValueType', 'SIGNED','Class', 'int16','Signed', [ 1;],'Factor', [ 1;],'Offset', [ 0;],'Min', [ -50;],'Max', [ 350;],'Units', 'degC','Comment', 'Temperature of the DC+ terminal','StartBit', [ 0;]),struct('Name', 'TemperatureDC2','Startbit', [ 0;],'SignalSize', [ 16;],'ByteOrder', 'LittleEndian','ValueType', 'SIGNED','Class', 'int16','Signed', [ 1;],'Factor', [ 1;],'Offset', [ 0;],'Min', [ -50;],'Max', [ 350;],'Units', 'degC','Comment', 'Temperature of the DC- terminal','StartBit', [ 16;]),struct('Name', 'TemperatureAC','Startbit', [ 0;],'SignalSize', [ 1;],'ByteOrder', 'LittleEndian','ValueType', 'UNSIGNED','Class', 'uint8','Signed', [ 0;],'Factor', [ 1;],'Offset', [ 0;],'Min', [ 0;],'Max', [ 1;],'Units', '','Comment', 'Overtemperature of the sensor on AC terminals','StartBit', [ 32;])}}
      settings: SourceProductName=Raptor
  Data : Outport  VectorParamsAs1DForOutWhenUnconnected=off
  wires:
  raptor_can_rxmsg/4 -> CANRxField2/1  "TemperatureAC"
  raptor_can_rxmsg/3 -> CANRxField1/1  "TemperatureDC2"
  raptor_can_rxmsg/2 -> CANRxField/1  "TemperatureDC1"
  Bus Creator/1 -> Data/1  "MsgName"
  CANRxField2/1 -> Bus Creator/4
  CANRxField1/1 -> Bus Creator/3
  CANRxField/1 -> Bus Creator/2
  CANRxMsgStatus/1 -> Bus Creator/1
  DiagEnbl/1 -> CANRxMsgStatus/1
  raptor_can_rxmsg/1 -> CANRxMsgStatus/2  "Age"

== system VCMGCM1962020b_v2/Fgnd/Sensors/CAN/CCS Interface/MsgName ==
  DiagEnbl : Inport
  Bus Creator : BusCreator  Inputs=2
  CANRxField : Blocks_lib/CANRxField  typ='double'  custom=on  custom_nam=[nam '---']  custom_units='---'
  CANRxMsgStatus : Blocks_lib/CANRxMsgStatus  samptime=samptime  custom=on  custom_nam=[nam '---']  msgnam=CCSEVSE_AC_ChargeInfo1
  Header : Blocks_lib/Header  width=Landscape  addtext=''
  raptor_can_rxmsg : Raptor_lib/CAN/raptor_can_rxmsg  canDefinition=struct('dbcFile', 'm2iev-api.dbc','message', 'EVSE_AC_ChargeInfo1','comment', 'EVSE_AC_ChargeInfo1','signals', {{'EVSEMaxCurrent'}},'enabled', [ 1;],'canBus', 'bus','messageID', [ 259;],'idMask', [ 2047;],'payloadMask', [],'payloadValue', [],'period', [ 0;],'mailbox', '''''','queueSize', [ 1;],'label', [ 1;],'ver', [ 2;],'showID', [ 0;],'showRaw', [ 0;],'fill', [ 0;],'editID', [ 0;],'signalOrder', [ 3;])  canBus=bus  mailbox=''  payloadMask=[]  payloadValue=[]  idMask=hex2dec('7FF')  queueSize=1  showID=0  label=1  fill=0  id=259  showRaw=0  showAge=1  signalOrder=3  signalInfo={{struct('Name', 'EVSEMaxCurrent','Startbit', [ 0;],'SignalSize', [ 16;],'ByteOrder', 'LittleEndian','ValueType', 'UNSIGNED','Class', 'uint16','Signed', [ 0;],'Factor', [ 0.05;],'Offset', [ 0;],'Min', [ 0;],'Max', [ 3276.75;],'Units', 'A','Comment', 'Maximum current EV may draw from EVSE','StartBit', [ 0;])}}
      settings: SourceProductName=Raptor
  Data : Outport  VectorParamsAs1DForOutWhenUnconnected=off
  wires:
  raptor_can_rxmsg/2 -> CANRxField/1  "EVSEMaxCurrent"
  Bus Creator/1 -> Data/1  "MsgName"
  CANRxField/1 -> Bus Creator/2
  CANRxMsgStatus/1 -> Bus Creator/1
  DiagEnbl/1 -> CANRxMsgStatus/1
  raptor_can_rxmsg/1 -> CANRxMsgStatus/2  "Age"

== system VCMGCM1962020b_v2/Fgnd/Sensors/CAN/Charger/ChgrCCSA ==
  DiagEnbl : Inport
  Bus Creator : BusCreator  Inputs=13
  CANRxField : Blocks_lib/CANRxField  typ='double'  custom=on  custom_nam=[nam '---']  custom_units='---'
  CANRxField{1..2,5..10} (8 alike) : Blocks_lib/CANRxField  typ='boolean'  custom=on  custom_nam=[nam '---']  custom_units='---'
  CANRxField11 : Blocks_lib/CANRxField  typ='uint8'  custom=on  custom_nam=[nam '---']  custom_units='---'
  CANRxField3 : Blocks_lib/CANRxField  typ='double'  custom=on  custom_nam=[nam '---']  custom_units='---'
  CANRxField4 : Blocks_lib/CANRxField  typ='double'  custom=on  custom_nam=[nam '---']  custom_units='---'
  CANRxMsgStatus : Blocks_lib/CANRxMsgStatus  samptime=samptime  custom=on  custom_nam=[nam '---']  msgnam=ChgrCCSA
  Header : Blocks_lib/Header  width=Landscape  addtext=''
  raptor_can_rxmsg : Raptor_lib/CAN/raptor_can_rxmsg  canDefinition=struct('dbcFile', 'Dilong Digital Charger_dbc file.dbc','message', 'CCSA','comment', 'Charger Control System (A)','signals', {{'Chrgr_Out_volt','Chrgr_Out_curr','Chrgr_internal_temp','Chrgr_hardware_protect','Chargr_temp_flag','Chrgr_input_volt_flag','Start_State_flag','Comm_Status_flag','S2_switch_status','Electronic_lock_status','Charging_Socket_Overtemp_Alarm','CC_Status_Alarm'}},'enabled', [ 1 1 1 1 1 1 1 1 1 1 1 1;],'scaled', [ 1 1 1 1 1 1 1 1 1 1 1 1;],'canBus', 'bus','messageID', [ 419385573;],'idMask', [ 536870911;],'payloadMask', [],'payloadValue', [],'period', [ 0;],'mailbox', '''''','queueSize', [ 1;],'label', [ 1;],'ver', [ 2;],'showID', [ 0;],'showRaw', [ 0;],'showRawMsg', [ 0;],'showAge', [ 1;],'fill', [ 0;],'editID', [ 0;],'signalOrder', [ 3;],'signalAscDes', [ 1;])  canBus=bus  mailbox=''  payloadMask=[]  payloadValue=[]  idMask=hex2dec('1FFFFFFF')  queueSize=1  showID=0  label=1  fill=0  id=419385573  showRaw=0  showAge=1  signalOrder=3  signalInfo={{struct('Name', 'Chrgr_Out_volt','Startbit', [ 0;],'SignalSize', [ 16;],'ByteOrder', 'BigEndian','ValueType', 'UNSIGNED','Class', 'uint16','Signed', [ 0;],'Factor', [ 0.1;],'Offset', [ 0;],'Min', [ 0;],'Max', [ 1320;],'Units', 'V','Comment', '','StartBit', [ 8;]),struct('Name', 'Chrgr_Out_curr','Startbit', [ 0;],'SignalSize', [ 16;],'ByteOrder', 'BigEndian','ValueType', 'UNSIGNED','Class', 'uint16','Signed', [ 0;],'Factor', [ 0.1;],'Offset', [ 0;],'Min', [ 0;],'Max', [ 350;],'Units', 'A','Comment', '','StartBit', [ 24;]),struct('Name', 'Chrgr_internal_temp','Startbit', [ 0;],'SignalSize', [ 8;],'ByteOrder', 'BigEndian','ValueType', 'UNSIGNED','Class', 'uint8','Signed', [ 0;],'Factor', [ 1;],'Offset', [ -40;],'Min', [ 0;],'Max', [ 300;],'Units', 'C','Comment', '','StartBit', [ 48;]),struct('Name', 'Chrgr_hardware_protect','Startbit', [ 0;],'SignalSize', [ 1;],'ByteOrder', 'BigEndian','ValueType', 'UNSIGNED','Class', 'uint8','Signed', [ 0;],'Factor', [ 1;],'Offset', [ 0;],'Min', [ 0;],'Max', [ 1;],'Units', 'enum','Comment', '','StartBit', [ 32;]),struct('Name', 'Chargr_temp_flag','Startbit', [ 0;],'SignalSize', [ 1;],'ByteOrder', 'BigEndian','ValueType', 'UNSIGNED','Class', 'uint8','Signed', [ 0;],'Factor', [ 1;],'Offset', [ 0;],'Min', [ 0;],'Max', [ 1;],'Units', 'enum','Comment', '','StartBit', [ 33;]),struct('Name', 'Chrgr_input_volt_flag','Startbit', [ 0;],'SignalSize', [ 1;],'ByteOrder', 'BigEndian','ValueType', 'UNSIGNED','Class', 'uint8','Signed', [ 0;],'Factor', [ 1;],'Offset', [ 0;],'Min', [ 0;],'Max', [ 1;],'Units', 'enum','Comment', '','StartBit', [ 34;]),struct('Name', 'Start_State_flag','Startbit', [ 0;],'SignalSize', [ 1;],'ByteOrder', 'BigEndian','ValueType', 'UNSIGNED','Class', 'uint8','Signed', [ 0;],'Factor', [ 1;],'Offset', [ 0;],'Min', [ 0;],'Max', [ 1;],'Units', 'enum','Comment', '','StartBit', [ 35;]),struct('Name', 'Comm_Status_flag','Startbit', [ 0;],'SignalSize', [ 1;],'ByteOrder', 'BigEndian','ValueType', 'UNSIGNED','Class', 'uint8','Signed', [ 0;],'Factor', [ 1;],'Offset', [ 0;],'Min', [ 0;],'Max', [ 1;],'Units', 'enum','Comment', '','StartBit', [ 36;]),struct('Name', 'S2_switch_status','Startbit', [ 0;],'SignalSize', [ 1;],'ByteOrder', 'BigEndian','ValueType', 'UNSIGNED','Class', 'uint8','Signed', [ 0;],'Factor', [ 1;],'Offset', [ 0;],'Min', [ 0;],'Max', [ 1;],'Units', 'enum','Comment', '','StartBit', [ 40;]),struct('Name', 'Electronic_lock_status','Startbit', [ 0;],'SignalSize', [ 2;],'ByteOrder', 'BigEndian','ValueType', 'UNSIGNED','Class', 'uint8','Signed', [ 0;],'Factor', [ 1;],'Offset', [ 0;],'Min', [ 0;],'Max', [ 1;],'Units', 'enum','Comment', '','StartBit', [ 41;]),struct('Name', 'Charging_Socket_Overtemp_Alarm','Startbit', [ 0;],'SignalSize', [ 1;],'ByteOrder', 'BigEndian','ValueType', 'UNSIGNED','Class', 'uint8','Signed', [ 0;],'Factor', [ 2;],'Offset', [ 0;],'Min', [ 0;],'Max', [ 1;],'Units', 'enum','Comment', '','StartBit', [ 43;]),struct('Name', 'CC_Status_Alarm','Startbit', [ 0;],'SignalSize', [ 1;],'ByteOrder', 'BigEndian','ValueType', 'UNSIGNED','Class', 'uint8','Signed', [ 0;],'Factor', [ 1;],'Offset', [ 0;],'Min', [ 0;],'Max', [ 1;],'Units', 'enum','Comment', '','StartBit', [ 44;])}}
      settings: SourceProductName=Raptor
  Data : Outport  VectorParamsAs1DForOutWhenUnconnected=off
  wires:
  Bus Creator/1 -> Data/1  "ChgrCCSA"
  raptor_can_rxmsg/2 -> CANRxField/1  "Chrgr_Out_volt"
  CANRxField5/1 -> Bus Creator/5
  CANRxField4/1 -> Bus Creator/4
  CANRxField3/1 -> Bus Creator/3
  CANRxField/1 -> Bus Creator/2
  CANRxMsgStatus/1 -> Bus Creator/1
  DiagEnbl/1 -> CANRxMsgStatus/1
  raptor_can_rxmsg/1 -> CANRxMsgStatus/2  "Age"
  raptor_can_rxmsg/3 -> CANRxField3/1  "Chrgr_Out_curr"
  raptor_can_rxmsg/4 -> CANRxField4/1  "Chrgr_internal_temp"
  raptor_can_rxmsg/5 -> CANRxField5/1  "Chrgr_hardware_protect"
  raptor_can_rxmsg/11 -> CANRxField11/1  "Electronic_lock_status"
  raptor_can_rxmsg/12 -> CANRxField10/1  "Charging_Socket_Overtemp_Alarm"
  raptor_can_rxmsg/13 -> CANRxField9/1  "CC_Status_Alarm"
  raptor_can_rxmsg/8 -> CANRxField6/1  "Start_State_flag"
  raptor_can_rxmsg/7 -> CANRxField2/1  "Chrgr_input_volt_flag"
  raptor_can_rxmsg/10 -> CANRxField8/1  "S2_switch_status"
  raptor_can_rxmsg/6 -> CANRxField1/1  "Chargr_temp_flag"
  raptor_can_rxmsg/9 -> CANRxField7/1  "Comm_Status_flag"
  CANRxField1/1 -> Bus Creator/6
  CANRxField2/1 -> Bus Creator/7
  CANRxField7/1 -> Bus Creator/9
  CANRxField8/1 -> Bus Creator/10
  CANRxField11/1 -> Bus Creator/11
  CANRxField10/1 -> Bus Creator/12
  CANRxField9/1 -> Bus Creator/13
  CANRxField6/1 -> Bus Creator/8

== system VCMGCM1962020b_v2/Fgnd/Sensors/CAN/Charger/ChgrCCSB ==
  DiagEnbl : Inport
  Bus Creator : BusCreator  Inputs=5
  CANRxField{,1,3..4} (4 alike) : Blocks_lib/CANRxField  typ='double'  custom=on  custom_nam=[nam '---']  custom_units='---'
  CANRxMsgStatus : Blocks_lib/CANRxMsgStatus  samptime=samptime  custom=on  custom_nam=[nam '---']  msgnam=ChgrCCSB
  Header : Blocks_lib/Header  width=Landscape  addtext=''
  raptor_can_rxmsg : Raptor_lib/CAN/raptor_can_rxmsg  canDefinition=struct('dbcFile', 'Dilong Digital Charger_dbc file.dbc','message', 'CCSB','comment', 'Charger Control System (B)','signals', {{'Input_volt_phase1','Input_curr_phase1','Input_volt_phase2','Input_curr_phase2'}},'enabled', [ 1 1 1 1;],'scaled', [ 1 1 1 1;],'canBus', 'bus','messageID', [ 419385829;],'idMask', [ 536870911;],'payloadMask', [],'payloadValue', [],'period', [ 0;],'mailbox', '''''','queueSize', [ 1;],'label', [ 1;],'ver', [ 2;],'showID', [ 0;],'showRaw', [ 0;],'showRawMsg', [ 0;],'showAge', [ 1;],'fill', [ 0;],'editID', [ 0;],'signalOrder', [ 3;],'signalAscDes', [ 1;])  canBus=bus  mailbox=''  payloadMask=[]  payloadValue=[]  idMask=hex2dec('1FFFFFFF')  queueSize=1  showID=0  label=1  fill=0  id=419385829  showRaw=0  showAge=1  signalOrder=3  signalInfo={{struct('Name', 'Input_volt_phase1','Startbit', [ 0;],'SignalSize', [ 16;],'ByteOrder', 'BigEndian','ValueType', 'UNSIGNED','Class', 'uint16','Signed', [ 0;],'Factor', [ 0.1;],'Offset', [ 0;],'Min', [ 0;],'Max', [ 132;],'Units', 'V','Comment', '','StartBit', [ 8;]),struct('Name', 'Input_curr_phase1','Startbit', [ 0;],'SignalSize', [ 16;],'ByteOrder', 'BigEndian','ValueType', 'UNSIGNED','Class', 'uint16','Signed', [ 0;],'Factor', [ 0.1;],'Offset', [ 0;],'Min', [ 0;],'Max', [ 35;],'Units', 'A','Comment', '','StartBit', [ 24;]),struct('Name', 'Input_volt_phase2','Startbit', [ 0;],'SignalSize', [ 16;],'ByteOrder', 'BigEndian','ValueType', 'UNSIGNED','Class', 'uint16','Signed', [ 0;],'Factor', [ 0.1;],'Offset', [ 0;],'Min', [ 0;],'Max', [ 132;],'Units', 'V','Comment', '','StartBit', [ 40;]),struct('Name', 'Input_curr_phase2','Startbit', [ 0;],'SignalSize', [ 16;],'ByteOrder', 'BigEndian','ValueType', 'UNSIGNED','Class', 'uint16','Signed', [ 0;],'Factor', [ 0.1;],'Offset', [ 0;],'Min', [ 0;],'Max', [ 35;],'Units', 'A','Comment', '','StartBit', [ 56;])}}
      settings: SourceProductName=Raptor
  Data : Outport  VectorParamsAs1DForOutWhenUnconnected=off
  wires:
  Bus Creator/1 -> Data/1  "ChgrCCSB"
  raptor_can_rxmsg/2 -> CANRxField/1  "Input_volt_phase1"
  CANRxField4/1 -> Bus Creator/4
  CANRxField3/1 -> Bus Creator/3
  CANRxField/1 -> Bus Creator/2
  CANRxMsgStatus/1 -> Bus Creator/1
  DiagEnbl/1 -> CANRxMsgStatus/1
  raptor_can_rxmsg/1 -> CANRxMsgStatus/2  "Age"
  raptor_can_rxmsg/3 -> CANRxField3/1  "Input_curr_phase1"
  raptor_can_rxmsg/4 -> CANRxField4/1  "Input_volt_phase2"
  raptor_can_rxmsg/5 -> CANRxField1/1  "Input_curr_phase2"
  CANRxField1/1 -> Bus Creator/5

== system VCMGCM1962020b_v2/Fgnd/Sensors/CAN/Charger/ChgrCCSC ==
  DiagEnbl : Inport
  Bus Creator : BusCreator  Inputs=3
  CANRxField : Blocks_lib/CANRxField  typ='double'  custom=on  custom_nam=[nam '---']  custom_units='---'
  CANRxField3 : Blocks_lib/CANRxField  typ='double'  custom=on  custom_nam=[nam '---']  custom_units='---'
  CANRxMsgStatus : Blocks_lib/CANRxMsgStatus  samptime=samptime  custom=on  custom_nam=[nam '---']  msgnam=ChgrCCSC
  Header : Blocks_lib/Header  width=Landscape  addtext=''
  raptor_can_rxmsg : Raptor_lib/CAN/raptor_can_rxmsg  canDefinition=struct('dbcFile', 'Dilong Digital Charger_dbc file.dbc','message', 'CCSC','comment', 'Charger Control System (C)','signals', {{'Input_volt_phase3','Input_curr_phase3'}},'enabled', [ 1 1;],'scaled', [ 1 1;],'canBus', 'bus','messageID', [ 419386085;],'idMask', [ 536870911;],'payloadMask', [],'payloadValue', [],'period', [ 0;],'mailbox', '''''','queueSize', [ 1;],'label', [ 1;],'ver', [ 2;],'showID', [ 0;],'showRaw', [ 0;],'showRawMsg', [ 0;],'showAge', [ 1;],'fill', [ 0;],'editID', [ 0;],'signalOrder', [ 3;],'signalAscDes', [ 1;])  canBus=bus  mailbox=''  payloadMask=[]  payloadValue=[]  idMask=hex2dec('1FFFFFFF')  queueSize=1  showID=0  label=1  fill=0  id=419386085  showRaw=0  showAge=1  signalOrder=3  signalInfo={{struct('Name', 'Input_volt_phase3','Startbit', [ 0;],'SignalSize', [ 16;],'ByteOrder', 'BigEndian','ValueType', 'UNSIGNED','Class', 'uint16','Signed', [ 0;],'Factor', [ 0.1;],'Offset', [ 0;],'Min', [ 0;],'Max', [ 132;],'Units', 'V','Comment', '','StartBit', [ 8;]),struct('Name', 'Input_curr_phase3','Startbit', [ 0;],'SignalSize', [ 16;],'ByteOrder', 'BigEndian','ValueType', 'UNSIGNED','Class', 'uint16','Signed', [ 0;],'Factor', [ 0.1;],'Offset', [ 0;],'Min', [ 0;],'Max', [ 35;],'Units', 'A','Comment', '','StartBit', [ 24;])}}
      settings: SourceProductName=Raptor
  Data : Outport  VectorParamsAs1DForOutWhenUnconnected=off
  wires:
  Bus Creator/1 -> Data/1  "ChgrCCSC"
  raptor_can_rxmsg/2 -> CANRxField/1  "Input_volt_phase3"
  CANRxField3/1 -> Bus Creator/3
  CANRxField/1 -> Bus Creator/2
  CANRxMsgStatus/1 -> Bus Creator/1
  DiagEnbl/1 -> CANRxMsgStatus/1
  raptor_can_rxmsg/1 -> CANRxMsgStatus/2  "Age"
  raptor_can_rxmsg/3 -> CANRxField3/1  "Input_curr_phase3"
